simulink model "BC1"  (R2021b)
settings: Solver=VariableStepAuto  StartTime=0.0  StopTime=10.0  RelTol=1e-3
values from neighbouring files (symbols this model uses):
  controlador = projetarControlador(planta)    [avaliaAS.m]    (also in avaliaBC1.m; avaliaBC2.m = projetarControladorPI(planta); avaliaCI.m; avaliaMalhaPura.m)
  planta = obterPlanta()    [avaliaAS.m]    (also in avaliaBC1.m; avaliaBC2.m; avaliaCI.m; avaliaMalhaPura.m)
settings Model: Creator=gagan  LastModifiedBy=emanu

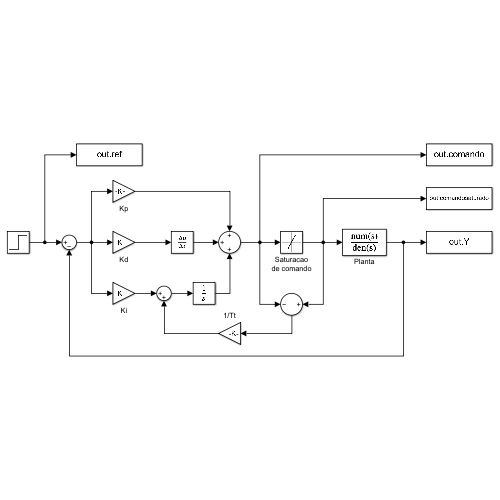
[thumbnail: Simulink's stored preview of the top-level diagram]
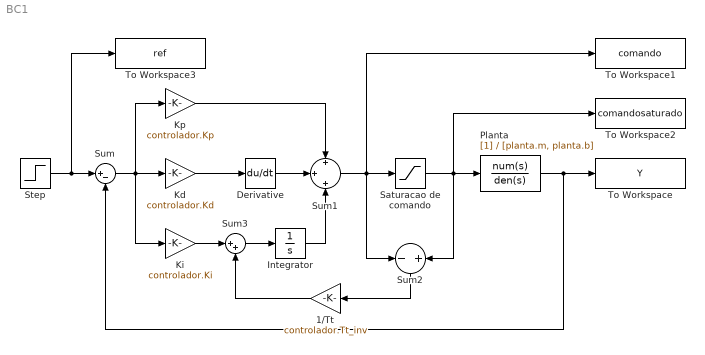
== system BC1 ==
  1/Tt : Gain  Gain=controlador.Tt_inv
  Derivative : Derivative
  Integrator : Integrator
  Kd : Gain  Gain=controlador.Kd
  Ki : Gain  Gain=controlador.Ki
  Kp : Gain  Gain=controlador.Kp
  Planta : TransferFcn  Denominator=[planta.m, planta.b]  ParameterTunability=Optimized
  Saturacao de comando : Saturate  UpperLimit=planta.comandoNominal  LowerLimit=-planta.comandoNominal
  Step : Step  SampleTime=0
  Sum : Sum  Inputs=|+-
  Sum1 : Sum  Inputs=+|+|+
  Sum2 : Sum  Inputs=-|+  OutDataTypeStr=Inherit: Keep LSB
  Sum3 : Sum  Inputs=|++
  To Workspace : ToWorkspace  VariableName=Y  SaveFormat=Structure With Time  SampleTime=-1
  To Workspace1 : ToWorkspace  VariableName=comando  SaveFormat=Structure With Time  SampleTime=-1
  To Workspace2 : ToWorkspace  VariableName=comandosaturado  SaveFormat=Structure With Time  SampleTime=-1
  To Workspace3 : ToWorkspace  VariableName=ref  SaveFormat=Structure With Time  SampleTime=-1
  wires:
  Sum/1 -> Ki/1, Kd/1, Kp/1
  Kp/1 -> Sum1/1
  Sum1/1 -> Saturacao de comando/1, To Workspace1/1, Sum2/1
  Saturacao de comando/1 -> To Workspace2/1, Sum2/2, Planta/1
  Planta/1 -> To Workspace/1, Sum/2
  Kd/1 -> Derivative/1
  Derivative/1 -> Sum1/2
  Integrator/1 -> Sum1/3
  Ki/1 -> Sum3/1
  Sum3/1 -> Integrator/1
  1/Tt/1 -> Sum3/2
  Sum2/1 -> 1/Tt/1
  Step/1 -> To Workspace3/1, Sum/1
